simulink model "stuPlutoTx"  (R2021a)
settings: Solver=VariableStepAuto  StartTime=0.0  StopTime=inf  FixedStep=1e-5  RelTol=1e-3
undefined symbols (not defined in the file or in its folder): designMultirateFIR, Fs, ip, usb
libraries: dspsrcs4 x2, plutoradiolib x1, dspmlti4 x1
settings Model: Creator=dm  LastModifiedBy=timingyang
settings SolverCC: AlgebraicLoopSolver=TrustRegion
settings ModelReferenceCC: EnableParallelModelReferenceBuilds=on

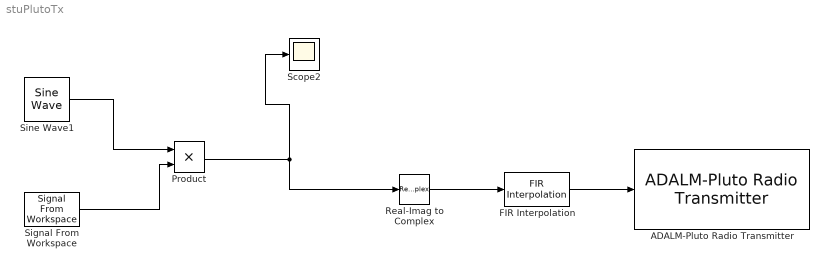
== system stuPlutoTx ==
  ADALM-Pluto Radio Transmitter : plutoradiolib/ADALM-Pluto Radio Transmitter  RadioID=usb:0  uri=ip:10.0.0.200  CenterFrequencySource=Dialog  CenterFrequency=915.432e6  GainSource=Dialog  Gain=0  ChannelMapping=1  BasebandSampleRate=1e6  UnderflowOutputPort=off  ShowAdvancedProperties=off  UseCustomFilter=off  filtPathRates=[737280000 11520000 3840000 1920000 960000 240000]  filtCoefficients=[-192 82 85 -215 228 -102 -110 290 -318 145 160 -426 471 -215 -238 633 -697 318 349 -923 1009 -457 -498 1309 -1423 640 693 -1812 1959 -876 -945 2458 -2647 1180 1268 -3290 3534 -1572 -1688 4375 -4698 2091 2247 -5836 6284 -2807 -3031 7918 -8588 3870 4225 -11182 12324 -5662 -6330 17255 -19735 9507 11312 -33568 43355 -25227 -42139 305542 305542 -42139 -25227 43355 -33568 11312 9507 -19735 17255 -6330 -5662 12324 -11182 4225 3870 -8588 7918 -3031 -2807 6284 -5836 2247 2091 -4698 4375 -1688 -1572 3534 -3290 1268 1180 -2647 2458 -945 -876 1959 -1812 693 640 -1423 1309 -498 -457 1009 -923 349 318 -697 633 -238 -215 471 -426 160 145 -318 290 -110 -102 228 -215 85 82 -192]  filtCoefficientSize=128  filtDecimInterpFactor=4  filtGain=-12  filtRFBandwidth=18000000  filterConfigStruct=struct()  DataSourceSelect=Input Port  DDSTone1Freq=5e3  DDSTone2Freq=10e3  DDSTone1Scale=0.5  DDSTone2Scale=0.25  DataTimeout=Inf  FrequencyCorrection=0  ENSMPinControlMode=None  BISTLoopbackMode=Disabled  BISTToneInject=Disabled  BISTSignalGen=PRBS  BISTToneFreq=Fs/32  BISTToneLevel=0
      settings: SourceProductBaseCode=PLUTO
  FIR Interpolation : dspmlti4/FIR Interpolation  FilterSource=Auto  PrivateCoeffs=0  h=designMultirateFIR(3,1)  L=10  FilterObject=FINTERP  InputProcessing=Columns as channels (frame based)  framing=Allow multirate processing  outputBufInitCond=0  roundingMode=Floor  overflowMode=off  firstCoeffDataTypeStr=Inherit: Same word length as input  firstCoeffMin=[]  firstCoeffMax=[]  firstCoeffLastDataTypeStr=Inherit: Same word length as input  outputDataTypeStr=Inherit: Same as accumulator  outputMin=[]  outputMax=[]  outputLastDataTypeStr=Inherit: Same as accumulator
  Product : Product  RndMeth=Zero
  Real-Imag to Complex : RealImagToComplex  Input=Real
  Scope2 : Scope
  Signal From Workspace : dspsrcs4/Signal From Workspace  X=txWave  Ts=1/100e3  nsamps=20000  OutputAfterFinalValue=Cyclic repetition  ignoreOrWarnInputAndFrameLengths=on  OutputFrames=off
  Sine Wave1 : dspsrcs4/Sine Wave  Amplitude=1  Frequency=10000  Phase=0  SampleMode=Discrete  OutComplex=Real  CompMethod=Table lookup  TableSize=Speed  SampleTime=1/100e3  SamplesPerFrame=20000  ResetState=Restart at time zero  OutputFrames=off  dataType=double  wordLen=16  udDataType=sfix(16)  fracBitsMode=Best precision  numFracBits=15  OutDataTypeStr=double  LastOutDataTypeStr=double
  wires:
  FIR Interpolation/1 -> ADALM-Pluto Radio Transmitter/1
  Real-Imag to Complex/1 -> FIR Interpolation/1
  Product/1 -> Real-Imag to Complex/1, Scope2/1
  Signal From Workspace/1 -> Product/2
  Sine Wave1/1 -> Product/1
